simulink model "CAD_test4_3"  (R2019a)
settings: Solver=VariableStepAuto  StartTime=0.0  StopTime=10.0  RelTol=1e-3
settings Model: Creator=83621  LastModifiedBy=83621

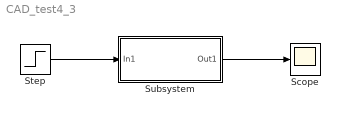
== system CAD_test4_3 ==
  Scope : Scope
  Step : Step  SampleTime=0
  Subsystem : Subsystem  mask(PIDControl){Kp=2, Ti=1, Td=2, N=20}
  wires:
  Step/1 -> Subsystem/1(In1)
  Subsystem/1(Out1) -> Scope/1

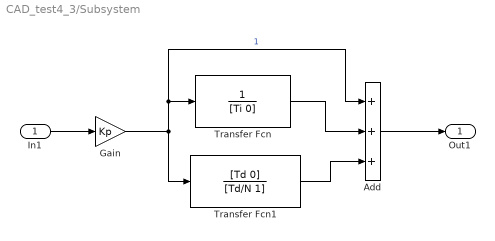
== system CAD_test4_3/Subsystem ==
  In1 : Inport
  Add : Sum  Inputs=3
  Gain : Gain  Gain=Kp
  Transfer Fcn : TransferFcn  Denominator=[Ti 0]
  Transfer Fcn1 : TransferFcn  Numerator=[Td 0]  Denominator=[Td/N 1]
  Out1 : Outport
  wires:
  In1/1 -> Gain/1
  Gain/1 -> Transfer Fcn1/1, Add/1, Transfer Fcn/1  "1"
  Transfer Fcn/1 -> Add/2
  Transfer Fcn1/1 -> Add/3
  Add/1 -> Out1/1
